simulink model "sl_subsys_fcncallerr4"  (Simulink 7.6)
settings: Solver=FixedStepDiscrete  StartTime=0.0  StopTime=10.0  FixedStep=1  RelTol=1e-3
Description:
  | Ambiguous execution order due to feedback of modified function-call output
  | 
  | The Chart is making the function-call [d1,d2]=f(), i.e., it is invoking f() and then
  | later using the values d1 and d2. When f() executes, it attempts to use the value B(Out2).
  | However, B does not execute when f() executes, thus creating an erroneous model.
settings Model: Creator=The MathWorks Inc.  CovMetricSettings=d  ExtModeAutoUpdateStatusClock=off
settings DataIOCC: SignalLoggingName=logsOut
settings OptimizationCC: BlockReduction=off  BooleanDataType=off  InlineInvariantSignals=on  InitFltsAndDblsToZero=on
settings DebuggingCC: SaveWithParameterizedLinksMsg=none  SignalResolutionControl=TryResolveAllWithWarning  SolverPrmCheckMsg=none  MultiTaskDSMMsg=warning  MultiTaskCondExecSysMsg=none
settings HardwareCC: TargetUnknown=on
settings SFSimCC: SimParseCustomCode=off
settings RTWCC: IncludeERTFirstTime=on
settings CodeAppCC: CustomSymbolStrFcn=$F$N$M
settings GRTTargetCC: TargetFcnLib=ansi_tfl_tmw.mat

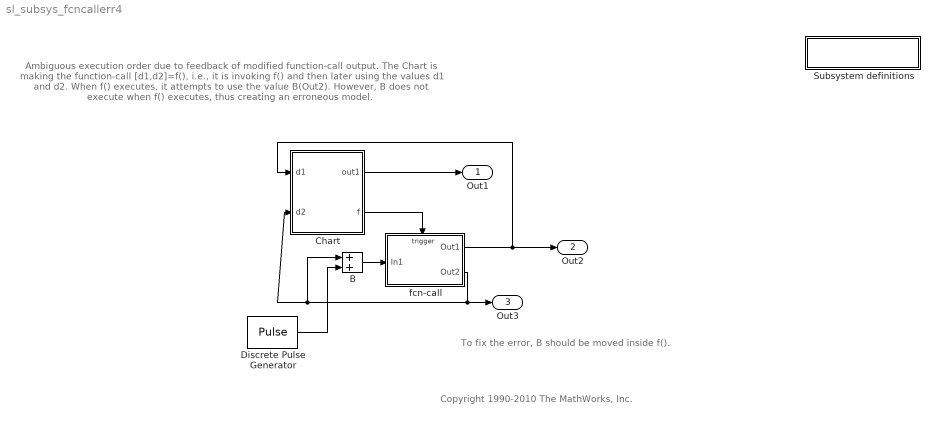
== system sl_subsys_fcncallerr4 ==
  note: Ambiguous execution order due to feedback of modified function-call output.
      |
      | The Chart is making the function-call [d1,d2]=f(), i.e., it is invoking f() and then
      | later using the values d1 and d2. When f() executes, it attempts to use the value B(Out2).
      | However, B does not execute when f() executes, thus creating an erroneous model.
  note: To fix the error, B should be moved inside f().
  note: Copyright 1990-2010 The MathWorks, Inc.
  " Subsystem definitions" : Subsystem
      settings: OpenFcn=helpview([matlabroot,'/toolbox/simulink/simdemos/simfeatures/html/sl_subsys_definitions.html']);
      mask Display: disp('Subsystem\ndefinitions')
  B : Sum  SaturateOnIntegerOverflow=on  InputSameDT=on  OutDataTypeStr=Inherit: Same as first input
  Chart : Stateflow chart  TreatAsAtomicUnit=on
  Discrete Pulse Generator : DiscretePulseGenerator
  fcn-call : Subsystem  TreatAsAtomicUnit=on
  Out1 : Outport
  Out2 : Outport  Port=2
  Out3 : Outport  Port=3
  wires:
  Chart/2(f) -> fcn-call/Trigger
  fcn-call/1(Out1) -> Out2/1, Chart/1(d1)
  fcn-call/2(Out2) -> Out3/1, B/1, Chart/2(d2)
  Chart/1(out1) -> Out1/1
  B/1 -> fcn-call/1(In1)
  Discrete Pulse Generator/1 -> B/2

== system sl_subsys_fcncallerr4/ Subsystem definitions ==

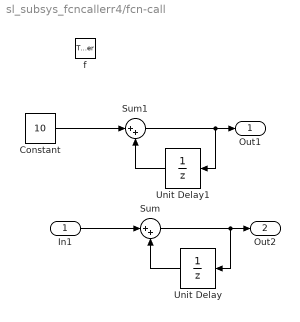
== system sl_subsys_fcncallerr4/fcn-call ==
  In1 : Inport
  f : TriggerPort  TriggerType=function-call  StatesWhenEnabling=reset
  Constant : Constant  Value=10
  Sum : Sum  Inputs=|++  SaturateOnIntegerOverflow=on  InputSameDT=on  OutDataTypeStr=Inherit: Same as first input
  Sum1 : Sum  Inputs=|++  SaturateOnIntegerOverflow=on  InputSameDT=on  OutDataTypeStr=Inherit: Same as first input
  Unit Delay : UnitDelay  SampleTime=-1
  Unit Delay1 : UnitDelay  SampleTime=-1
  Out1 : Outport
  Out2 : Outport  Port=2
  wires:
  In1/1 -> Sum/1
  Unit Delay/1 -> Sum/2
  Sum/1 -> Unit Delay/1, Out2/1
  Unit Delay1/1 -> Sum1/2
  Sum1/1 -> Unit Delay1/1, Out1/1
  Constant/1 -> Sum1/1

== stateflow chart Chart ==
  state one/
    entry:f;out1=d1+d2;
  state two/
    entry: f;out1=d1-d2;
  one -> two
  two -> one
  (default) -> one
  data: d1 input double; d2 input double; out1 output double; out local double
  events: f output FUNCTION_CALL_EVENT
